simulink model "modelo_elser"  (R2015a)
settings: Solver=ode45  StartTime=0.0  StopTime=10.0  RelTol=1e-3
values from neighbouring files (symbols this model uses):
  C = 8.0e-1    (= 0.8)    [var_elser.m]
  K = 3.27e4    (= 32700)    [var_elser.m]
  Kb = 1.469e-1    (= 0.1469)    [var_elser.m]
  Kd = 0.007    [var_elser.m]
  KH = 3.336e6    (= 3336000)    [var_elser.m]
  Ki = 4.129    [var_elser.m]
  KL = 3.303e6    (= 3303000)    [var_elser.m]
  Kp = 2.915    [var_elser.m]
  KT = 1.470e-1    (= 0.147)    [var_elser.m]
  La = 8.2e-4    (= 0.00082)    [var_elser.m]
  M = 1.261    [var_elser.m]
  n = 0.001    [var_elser.m]
  p = 0.003    [var_elser.m]
  Ra = 1.03    [var_elser.m]
undefined symbols (not defined in the file or in its folder): CE, CH, JE, Kt
libraries: simulink x1
settings Model: Creator=11802972  LastModifiedBy=11802972

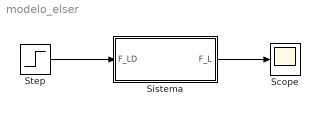
== system modelo_elser ==
  Scope : Scope
  "Sistema " : Subsystem
  Step : Step  Time=0  SampleTime=0
  wires:
  "Sistema "/1(F_L) -> Scope/1
  Step/1 -> "Sistema "/1(F_LD)

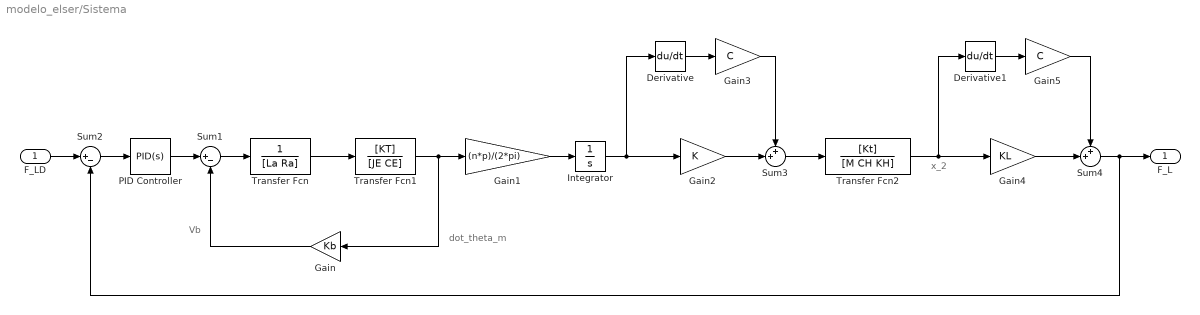
== system modelo_elser/Sistema  ==
  note: x_2
  note: dot_theta_m
  note: Vb
  F_LD : Inport
  Derivative : Derivative
  Derivative1 : Derivative
  Gain : Gain  Gain=Kb
  Gain1 : Gain  Gain=(n*p)/(2*pi)
  Gain2 : Gain  Gain=K
  Gain3 : Gain  Gain=C
  Gain4 : Gain  Gain=KL
  Gain5 : Gain  Gain=C
  Integrator : Integrator
  PID Controller : simulink/Continuous/PID Controller  Controller=PID  TimeDomain=Continuous-time  SampleTime=-1  IntegratorMethod=Forward Euler  FilterMethod=Forward Euler  Form=Parallel  UseFilter=on  ControllerParametersSource=internal  P=Kp  I=Ki  D=Kd  N=100  InitialConditionSource=internal  InitialConditionForIntegrator=0  InitialConditionForFilter=0  ExternalReset=none  LimitOutput=off  UpperSaturationLimit=inf  LowerSaturationLimit=-inf  LinearizeAsGain=on  AntiWindupMode=none  Kb=1  TrackingMode=off  Kt=1  PParamMin=[]  PParamMax=[]  IParamMin=[]  IParamMax=[]  DParamMin=[]  DParamMax=[]  NParamMin=[]  NParamMax=[]  KbParamMin=[]  KbParamMax=[]  KtParamMin=[]  KtParamMax=[]  POutMin=[]  POutMax=[]  IOutMin=[]  IOutMax=[]  DOutMin=[]  DOutMax=[]  NOutMin=[]  NOutMax=[]  KbOutMin=[]  KbOutMax=[]  KtOutMin=[]  KtOutMax=[]  IntegratorOutMin=[]  IntegratorOutMax=[]  FilterOutMin=[]  FilterOutMax=[]  SumOutMin=[]  SumOutMax=[]  SumI1OutMin=[]  SumI1OutMax=[]  SumI2OutMin=[]  SumI2OutMax=[]  SumI3OutMin=[]  SumI3OutMax=[]  SumDOutMin=[]  SumDOutMax=[]  SaturationOutMin=[]  SaturationOutMax=[]  IntegratorContinuousStateAttributes=''  IntegratorStateMustResolveToSignalObject=off  IntegratorRTWStateStorageClass=Auto  FilterContinuousStateAttributes=''  FilterStateMustResolveToSignalObject=off  FilterRTWStateStorageClass=Auto  DifferentiatorICPrevScaledInput=0  DifferentiatorOutMin=[]  DifferentiatorOutMax=[]
  Sum1 : Sum  Inputs=|+-
  Sum2 : Sum  Inputs=|+-
  Sum3 : Sum  Inputs=++|
  Sum4 : Sum  Inputs=++|
  Transfer Fcn : TransferFcn  Denominator=[La Ra]
  Transfer Fcn1 : TransferFcn  Numerator=[KT]  Denominator=[JE CE]
  Transfer Fcn2 : TransferFcn  Numerator=[Kt]  Denominator=[M CH KH]
  F_L : Outport
  wires:
  F_LD/1 -> Sum2/1
  Sum2/1 -> PID Controller/1
  PID Controller/1 -> Sum1/1
  Gain/1 -> Sum1/2
  Sum1/1 -> Transfer Fcn/1
  Transfer Fcn/1 -> Transfer Fcn1/1
  Transfer Fcn1/1 -> Gain1/1, Gain/1
  Gain1/1 -> Integrator/1
  Integrator/1 -> Gain2/1, Derivative/1
  Derivative/1 -> Gain3/1
  Gain3/1 -> Sum3/1
  Gain2/1 -> Sum3/2
  Sum3/1 -> Transfer Fcn2/1
  Derivative1/1 -> Gain5/1
  Transfer Fcn2/1 -> Derivative1/1, Gain4/1
  Gain5/1 -> Sum4/1
  Gain4/1 -> Sum4/2
  Sum4/1 -> F_L/1, Sum2/2
